simulink model "GDFLIB_FilterMA_BAM_F16"  (Simulink 7.3)
settings: Solver=ode45  StartTime=0.0  StopTime=10.0  RelTol=1e-3
undefined symbols (not defined in the file): u16NSamples
settings Model: Creator=RE004C  LastModifiedBy=RE004C
settings HardwareCC: ProdIntDivRoundTo=Zero  ProdEndianess=BigEndian  ProdHWDeviceType=Freescale->32-bit PowerPC

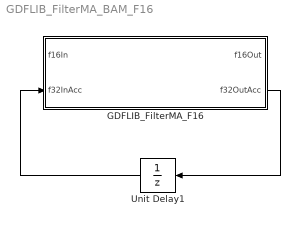
== system GDFLIB_FilterMA_BAM_F16 ==
  GDFLIB_FilterMA_F16 : Subsystem  mask(GDFLIB_FilterMA_F16){u16NSamples=u16NSamples}
      mask help: Bit accurate model of recursive form moving average filter. All parameters as well as input and output are 16bit integers.
      mask init:
      | pos = get_param(gcb, 'Position');width = pos(3) - pos(1); height = pos(4) - pos(2);tX=width/2;tY=height*0.9;
      mask Display:
      | color('black');
      | port_label('input',1,'f16In');
      | port_label('input',2,'f32InAcc');
      | port_label('output',1,'f16Out');
      | port_label('output',2,'f32OutAcc');
      | color('black');
      | disp('GDFLIB_FilterMA_F16');
      | color('blue');
      | text(tX,tY, 'BAM', 'horizontalAlignment', 'center');
  Unit Delay1 : UnitDelay  SampleTime=-1
  wires:
  GDFLIB_FilterMA_F16/2(f32OutAcc) -> Unit Delay1/1
  Unit Delay1/1 -> GDFLIB_FilterMA_F16/2(f32InAcc)

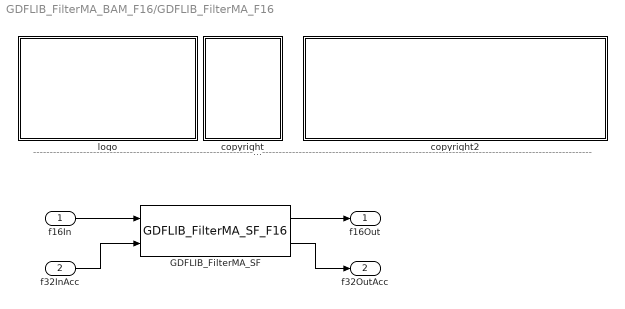
== system GDFLIB_FilterMA_BAM_F16/GDFLIB_FilterMA_F16 ==
  note: ---------------------------------------------------------------------------------------------------------------------------------------------------------------------------------------------------
  f16In : Inport  OutDataType=fixdt(1, 16)  OutScaling=2^0
  f32InAcc : Inport  Port=2  OutDataType=fixdt(1, 16)  OutScaling=2^0
  GDFLIB_FilterMA_SF : S-Function  FunctionName=GDFLIB_FilterMA_SF_F16  Parameters=u16NSamples  EnableBusSupport=off
  copyright : Subsystem
      mask Display: text(10,90,'FILE:');text(10,75,'DESRIPTION:')text(10,60,'COPYRIGHT:')text(10,45,'VERSION:')text(10,30,'DATE:')
  copyright2 : Subsystem
      mask Display: text(10,90,'GDFLIB_FilterMA_BAM_F16.mdl');text(10,75,'Recursive form moving average filter.');text(10,60,'Freescale')text(10,45,'0.1');text(10,30,'16-Jan-2012');
  logo : Subsystem
      mask Display: image(imread('logo.jpg'))
  f16Out : Outport  OutDataType=fixdt(1, 16)  OutScaling=2^0
  f32OutAcc : Outport  Port=2  OutDataType=fixdt(1, 16)  OutScaling=2^0
  wires:
  f16In/1 -> GDFLIB_FilterMA_SF/1
  GDFLIB_FilterMA_SF/1 -> f16Out/1
  GDFLIB_FilterMA_SF/2 -> f32OutAcc/1
  f32InAcc/1 -> GDFLIB_FilterMA_SF/2

== system GDFLIB_FilterMA_BAM_F16/GDFLIB_FilterMA_F16/copyright ==

== system GDFLIB_FilterMA_BAM_F16/GDFLIB_FilterMA_F16/copyright2 ==

== system GDFLIB_FilterMA_BAM_F16/GDFLIB_FilterMA_F16/logo ==
